simulink model "SimulationANTSMC"  (R2020b)
settings: Solver=ode3  StartTime=0.0  StopTime=100  FixedStep=0.001  RelTol=1e-6  EnableMultiTasking=on
model workspace (MAT data in the model file):
  time = 1
values from neighbouring files (symbols this model uses):
  beta = 2*x(3)/(1+x(3))    [GA_init.m]
  epstar = x(9)    [GA_init.m]
  g0 = x(5)    [GA_init.m]
  g1 = x(6)    [GA_init.m]
  g2 = x(7)    [GA_init.m]
  g3 = x(8)    [GA_init.m]
  gamma = x(3)    [GA_init.m]
  kappa = x(11)    [GA_init.m]
  landa = x(1)    [GA_init.m]
  nu = x(2)    [GA_init.m]
  vu = x(4)    [GA_init.m]
(part 16 of 18)

== matlab function SimulationANTSMC/Subsystem/S manifold ==
  data: despar input; e input; edot input; z1 output; z2 output; z3 output; z4 output; z5 output; z6 output
function [z1 ,z2, z3, z4, z5 ,z6]    = fcn(despar,e,edot)
%  1  2  3  4    5    6
% [g0,g1,g2,g3,gamma,beta]'
z1=despar(1)*((abs(e(1)))^despar(5))*sign(e(1))+despar(2)*e(1)+...
    despar(3)*(e(1)^3)+despar(4)*despar(6)*((abs(edot(1)))^(despar(6)))*sign(edot(1));

z2=despar(1)*((abs(e(2)))^despar(5))*sign(e(2))+despar(2)*e(2)+...
    despar(3)*(e(2)^3)+despar(4)*despar(6)*((abs(edot(2)))^(despar(6)))*sign(edot(2));

z3=despar(1)*((abs(e(3)))^despar(5))*sign(e(3))+despar(2)*e(3)+...
    despar(3)*(e(3)^3)+despar(4)*despar(6)*((abs(edot(3)))^(despar(6)))*sign(edot(3));

z4=despar(1)*((abs(e(4)))^despar(5))*sign(e(4))+despar(2)*e(4)+...
    despar(3)*(e(4)^3)+despar(4)*despar(6)*((abs(edot(4)))^(despar(6)))*sign(edot(4));

z5=despar(1)*((abs(e(5)))^despar(5))*sign(e(5))+despar(2)*e(5)+...
    despar(3)*(e(5)^3)+despar(4)*despar(6)*((abs(edot(5)))^(despar(6)))*sign(edot(5));

z6=despar(1)*((abs(e(6)))^despar(5))*sign(e(6))+despar(2)*e(6)+...
    despar(3)*(e(6)^3)+despar(4)*despar(6)*((abs(edot(6)))^(despar(6)))*sign(edot(6));
